simulink model "simulation"  (R2022b)
settings: Solver=ode4  StartTime=0  StopTime=Tend  FixedStep=Ts  RelTol=1e-3
values from neighbouring files (symbols this model uses):
  K1 = Kvec{1}    [main.m]
  K2 = Kvec{2}    [main.m]
  K3 = Kvec{3}    [main.m]
  K4 = Kvec{4}    [main.m]
  K5 = Kvec{5}    [main.m]
  K6 = Kvec{6}    [main.m]
  L = 2.8    [main.m]
  tau = 0.1    [main.m]
  v0 = vx0*cos(yaw0) + vy0*sin(yaw0)    [main.m]    (also in reference_data.mat = 7)
  x0 = egoVehicle.Position(1)    [main.m]    (also in reference_data.mat = -97.7)
  y0 = egoVehicle.Position(2)    [main.m]    (also in reference_data.mat = -2.1)
  yaw0 = deg2rad(egoVehicle.Yaw)    [main.m]    (also in reference_data.mat = 0)
libraries: simulink x1
settings Model: Creator=ludovicaperroni  LastModifiedBy=ludovicaperroni

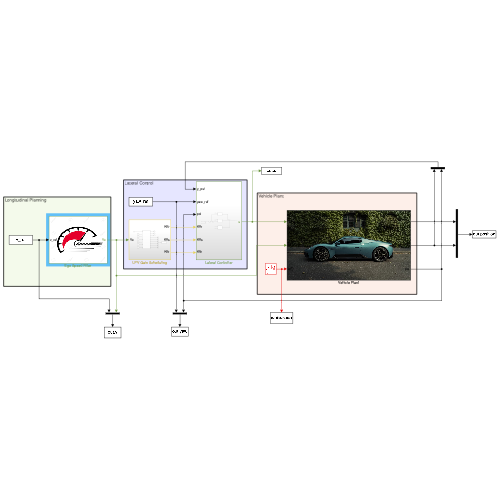
[thumbnail: Simulink's stored preview of the top-level diagram]
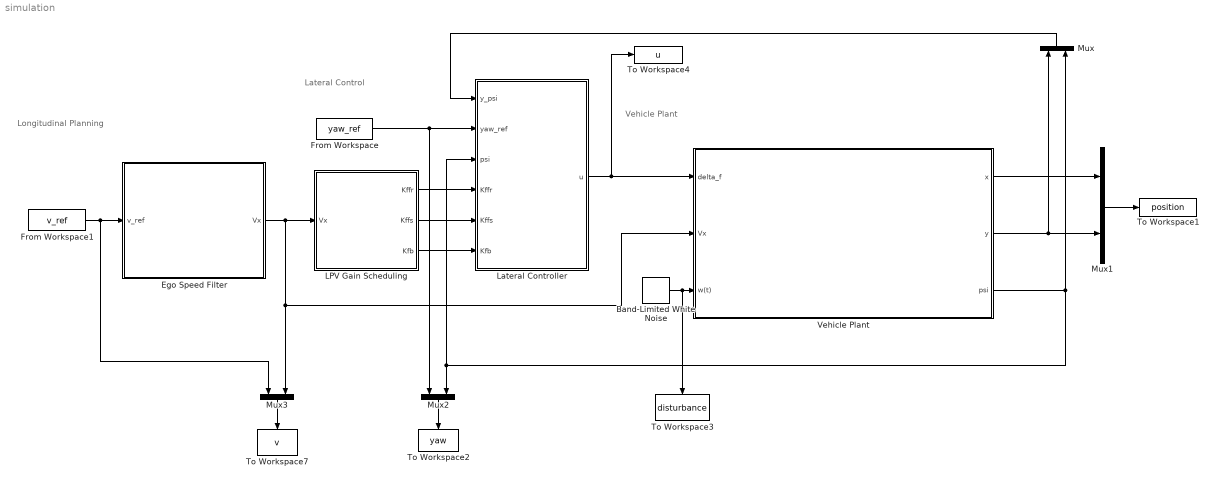
== system simulation ==
  note: Vehicle Plant
  note: Lateral Control
  note: Longitudinal Planning
  Band-Limited White Noise : simulink/Sources/Band-Limited White Noise  Cov=[0.001]  Ts=0.1  seed=[23341]
  Ego Speed Filter : Subsystem
      mask Display: image('/Users/ludovicaperroni/Desktop/Vehicle 2-Gagliardi/Vehicle2/project/immagini_simulink/speed.png'); % Use "Edit Image" on toolstrip to change.
  From Workspace : FromWorkspace  VariableName=yaw_ref
  From Workspace1 : FromWorkspace  VariableName=v_ref
  LPV Gain Scheduling : Subsystem
  Lateral Controller : Subsystem
  Mux{,1..3} (4 alike) : Mux  Inputs=2
  To Workspace1 : ToWorkspace  VariableName=position  SaveFormat=Timeseries  SampleTime=0.01
  To Workspace2 : ToWorkspace  VariableName=yaw  SaveFormat=Timeseries  SampleTime=0.01
  To Workspace3 : ToWorkspace  VariableName=disturbance  SaveFormat=Timeseries  SampleTime=0.01
  To Workspace4 : ToWorkspace  VariableName=u  SaveFormat=Timeseries  SampleTime=0.01
  To Workspace7 : ToWorkspace  VariableName=v  SaveFormat=Timeseries  SampleTime=0.01
  Vehicle Plant : Subsystem
      mask Display: image('/Users/ludovicaperroni/Desktop/Vehicle 2-Gagliardi/Vehicle2/project/immagini_simulink/vehicle.jpg'); % Use "Edit Image" on toolstrip to change.
  wires:
  Lateral Controller/1(u) -> To Workspace4/1, Vehicle Plant/1(delta_f)
  Ego Speed Filter/1(Vx) -> Vehicle Plant/2(Vx), Mux3/2, LPV Gain Scheduling/1(Vx)
  Band-Limited White Noise/1 -> To Workspace3/1, Vehicle Plant/3(w(t))
  LPV Gain Scheduling/2(Kffs) -> Lateral Controller/5(Kffs)
  LPV Gain Scheduling/3(Kfb) -> Lateral Controller/6(Kfb)
  LPV Gain Scheduling/1(Kffr) -> Lateral Controller/4(Kffr)
  Vehicle Plant/1(x) -> Mux1/1
  Vehicle Plant/2(y) -> Mux1/2, Mux/1
  Mux/1 -> Lateral Controller/1(y_psi)
  From Workspace/1 -> Lateral Controller/2(yaw_ref), Mux2/1
  Mux1/1 -> To Workspace1/1
  Vehicle Plant/3(psi) -> Mux2/2, Lateral Controller/3(psi), Mux/2
  From Workspace1/1 -> Ego Speed Filter/1(v_ref), Mux3/1
  Mux2/1 -> To Workspace2/1
  Mux3/1 -> To Workspace7/1

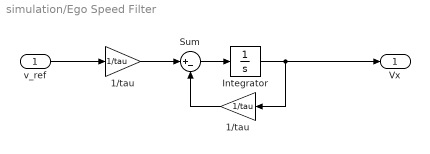
== system simulation/Ego Speed Filter ==
  v_ref : Inport
  1/tau : Gain  Gain=1/tau  SaturateOnIntegerOverflow=on
  "1/tau " : Gain  Gain=1/tau  SaturateOnIntegerOverflow=on
  Integrator : Integrator  InitialCondition=v0
  Sum : Sum  Inputs=|+-  SaturateOnIntegerOverflow=on
  Vx : Outport
  wires:
  1/tau/1 -> Sum/1
  Sum/1 -> Integrator/1
  Integrator/1 -> Vx/1, "1/tau "/1
  "1/tau "/1 -> Sum/2
  v_ref/1 -> 1/tau/1

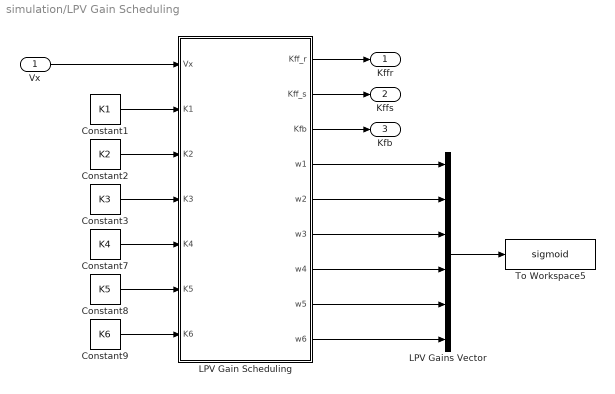
== system simulation/LPV Gain Scheduling ==
  Vx : Inport
  Constant1 : Constant  Value=K1
  Constant2 : Constant  Value=K2
  Constant3 : Constant  Value=K3
  Constant7 : Constant  Value=K4
  Constant8 : Constant  Value=K5
  Constant9 : Constant  Value=K6
  LPV Gain Scheduling : MATLAB Function  TreatAsAtomicUnit=on
  LPV Gains Vector : Mux  Inputs=6
  To Workspace5 : ToWorkspace  VariableName=sigmoid  SaveFormat=Timeseries  SampleTime=-1
  Kffr : Outport
  Kffs : Outport  Port=2
  Kfb : Outport  Port=3
  wires:
  Vx/1 -> LPV Gain Scheduling/1(Vx)
  Constant3/1 -> LPV Gain Scheduling/4(K3)
  LPV Gain Scheduling/5(w2) -> LPV Gains Vector/2
  Constant7/1 -> LPV Gain Scheduling/5(K4)
  LPV Gain Scheduling/4(w1) -> LPV Gains Vector/1
  LPV Gain Scheduling/7(w4) -> LPV Gains Vector/4
  Constant2/1 -> LPV Gain Scheduling/3(K2)
  LPV Gain Scheduling/8(w5) -> LPV Gains Vector/5
  Constant8/1 -> LPV Gain Scheduling/6(K5)
  LPV Gains Vector/1 -> To Workspace5/1
  Constant1/1 -> LPV Gain Scheduling/2(K1)
  LPV Gain Scheduling/9(w6) -> LPV Gains Vector/6
  Constant9/1 -> LPV Gain Scheduling/7(K6)
  LPV Gain Scheduling/6(w3) -> LPV Gains Vector/3
  LPV Gain Scheduling/1(Kff_r) -> Kffr/1
  LPV Gain Scheduling/2(Kff_s) -> Kffs/1
  LPV Gain Scheduling/3(Kfb) -> Kfb/1

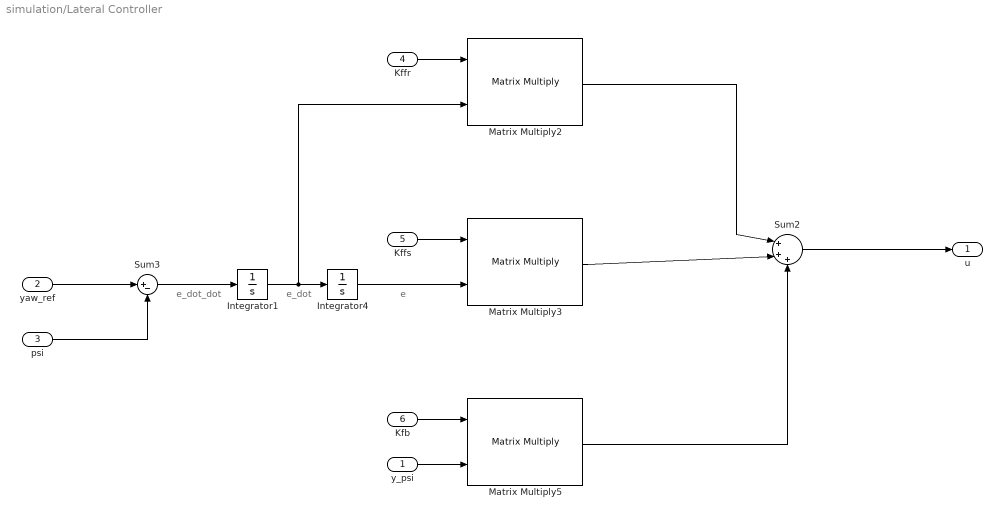
== system simulation/Lateral Controller ==
  note: e
  note: e_dot
  note: e_dot_dot
  y_psi : Inport
  yaw_ref : Inport  Port=2
  psi : Inport  Port=3
  Kffr : Inport  Port=4
  Kffs : Inport  Port=5
  Kfb : Inport  Port=6
  Integrator1 : Integrator
  Integrator4 : Integrator
  Matrix Multiply2 : Product  Multiplication=Matrix(*)
  Matrix Multiply3 : Product  Multiplication=Matrix(*)
  Matrix Multiply5 : Product  Multiplication=Matrix(*)
  Sum2 : Sum  Inputs=|+++
  Sum3 : Sum  Inputs=|+-
  u : Outport
  wires:
  Integrator1/1 -> Integrator4/1, Matrix Multiply2/2
  y_psi/1 -> Matrix Multiply5/2
  Sum2/1 -> u/1
  yaw_ref/1 -> Sum3/1
  Matrix Multiply3/1 -> Sum2/2
  Integrator4/1 -> Matrix Multiply3/2
  psi/1 -> Sum3/2
  Kffs/1 -> Matrix Multiply3/1
  Kffr/1 -> Matrix Multiply2/1
  Matrix Multiply2/1 -> Sum2/1
  Sum3/1 -> Integrator1/1
  Kfb/1 -> Matrix Multiply5/1
  Matrix Multiply5/1 -> Sum2/3

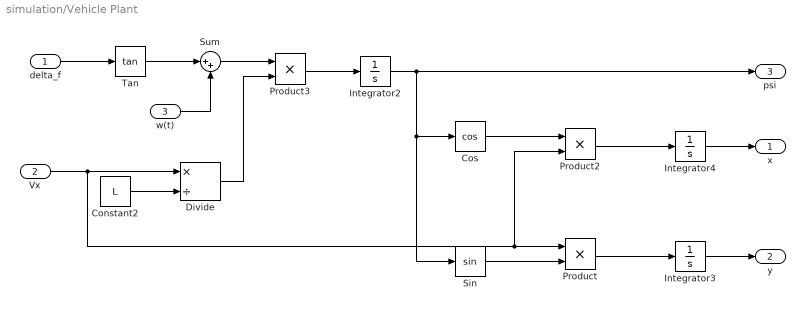
== system simulation/Vehicle Plant ==
  delta_f : Inport
  Vx : Inport  Port=2
  w(t) : Inport  Port=3
  Constant2 : Constant  Value=L
  Cos : Trigonometry  Operator=cos
  Divide : Product  Inputs=*/
  Integrator2 : Integrator  InitialCondition=yaw0
  Integrator3 : Integrator  InitialCondition=y0
  Integrator4 : Integrator  InitialCondition=x0
  Product : Product
  Product2 : Product
  Product3 : Product
  Sin : Trigonometry
  Sum : Sum  Inputs=|++
  Tan : Trigonometry  Operator=tan
  x : Outport  VectorParamsAs1DForOutWhenUnconnected=off
  y : Outport  Port=2  VectorParamsAs1DForOutWhenUnconnected=off
  psi : Outport  Port=3  VectorParamsAs1DForOutWhenUnconnected=off
  wires:
  Vx/1 -> Product2/2, Product/1, Divide/1
  delta_f/1 -> Tan/1
  Cos/1 -> Product2/1
  Integrator2/1 -> psi/1, Cos/1, Sin/1
  Product/1 -> Integrator3/1
  Constant2/1 -> Divide/2
  Sin/1 -> Product/2
  Product2/1 -> Integrator4/1
  Divide/1 -> Product3/2
  Product3/1 -> Integrator2/1
  Sum/1 -> Product3/1
  Integrator4/1 -> x/1
  Integrator3/1 -> y/1
  Tan/1 -> Sum/1
  w(t)/1 -> Sum/2

== matlab function simulation/LPV Gain Scheduling/LPV Gain Scheduling ==
  data: Vx input; K1 input; Kff_r output; Kff_s output; Kfb output; w1 output; w2 output; w3 output; w4 output; w5 output; w6 output; K2 input; K3 input; K4 input; K5 input; K6 input
function [Kff_r,Kff_s,Kfb,w1,w2,w3,w4,w5,w6] = fcn(Vx,K1,K2,K3,K4,K5,K6)
% fcn
% -------------------------------------------------------------------------
% LPV gain scheduling basato su:
% 1) attivazione smooth delle regioni di velocita'
% 2) interpolazione locale tra i due vertici di ciascun intervallo
% 3) combinazione pesata dei guadagni regionali
%
% INPUT:
%   Vx          velocita' corrente
%   K1...K6     guadagni dei 6 intervalli, ciascuno nel formato:
%               [K_low(1:4)  K_high(1:4)]
%
% OUTPUT:
%   Kff_r       primo coefficiente del guadagno totale
%   Kff_s       secondo coefficiente del guadagno totale
%   Kfb         ultimi due coefficienti del guadagno totale [1x2]
%   w1...w6     pesi smooth delle 6 regioni
% -------------------------------------------------------------------------

    %% Parametro che regola la pendenza delle sigmoidi
    beta = 10;

    %% Soglie di velocita' dei 6 intervalli
    v1 = 0.0;
    v2 = 1.2;
    v3 = 2.4;
    v4 = 3.6;
    v5 = 4.8;
    v6 = 6.0;
    v7 = 7.0;

    %% Pesi smooth delle regioni
    % Ogni regione e' ottenuta come differenza di funzioni logistiche
    s12 = 1/(1 + exp(-beta*(Vx - v2)));
    s23 = 1/(1 + exp(-beta*(Vx - v3)));
    s34 = 1/(1 + exp(-beta*(Vx - v4)));
    s45 = 1/(1 + exp(-beta*(Vx - v5)));
    s56 = 1/(1 + exp(-beta*(Vx - v6)));
    s67 = 1/(1 + exp(-beta*(Vx - v7)));

    w1 = 1 - s12;
    w2 = s12 - s23;
    w3 = s23 - s34;
    w4 = s34 - s45;
    w5 = s45 - s56;
    w6 = s56 - s67;

    %% Estrazione guadagni ai vertici dei 6 intervalli
    % Ogni Ki = [K_low(1:4)  K_high(1:4)]

    K1_low  = K1(1:4);   K1_high  = K1(5:8);
    K2_low  = K2(1:4);   K2_high  = K2(5:8);
    K3_low  = K3(1:4);   K3_high  = K3(5:8);
    K4_low  = K4(1:4);   K4_high  = K4(5:8);
    K5_low  = K5(1:4);   K5_high  = K5(5:8);
    K6_low  = K6(1:4);   K6_high  = K6(5:8);

    %% Interpolazione locale dentro ogni intervallo
    % La velocita' viene limitata al range locale per evitare extrapolazioni

    % Intervallo 1: [0, 1.2]
    Vloc1 = min(max(Vx,v1),v2);
    a1 = (Vloc1 - v1)/(v2 - v1);
    b1 = 1 - a1;

    % Intervallo 2: [1.2, 2.4]
    Vloc2 = min(max(Vx,v2),v3);
    a2 = (Vloc2 - v2)/(v3 - v2);
    b2 = 1 - a2;

    % Intervallo 3: [2.4, 3.6]
    Vloc3 = min(max(Vx,v3),v4);
    a3 = (Vloc3 - v3)/(v4 - v3);
    b3 = 1 - a3;

    % Intervallo 4: [3.6, 4.8]
    Vloc4 = min(max(Vx,v4),v5);
    a4 = (Vloc4 - v4)/(v5 - v4);
    b4 = 1 - a4;

    % Intervallo 5: [4.8, 6.0]
    Vloc5 = min(max(Vx,v5),v6);
    a5 = (Vloc5 - v5)/(v6 - v5);
    b5 = 1 - a5;

    % Intervallo 6: [6.0, 7.0]
    Vloc6 = min(max(Vx,v6),v7);
    a6 = (Vloc6 - v6)/(v7 - v6);
    b6 = 1 - a6;

    %% Guadagno interpolato per ciascuna regione
    Kreg1 = b1*K1_low + a1*K1_high;
    Kreg2 = b2*K2_low + a2*K2_high;
    Kreg3 = b3*K3_low + a3*K3_high;
    Kreg4 = b4*K4_low + a4*K4_high;
    Kreg5 = b5*K5_low + a5*K5_high;
    Kreg6 = b6*K6_low + a6*K6_high;

    %% Guadagno LPV complessivo
    Ktot = w1*Kreg1 + w2*Kreg2 + w3*Kreg3 + ...
           w4*Kreg4 + w5*Kreg5 + w6*Kreg6;

    %% Uscite separate
    Kff_r = Ktot(1);
    Kff_s = Ktot(2);
    Kfb   = Ktot(3:4)';

end
